simulink model "MathematicalOperations"  (R2026a)
settings: Solver=VariableStepAuto
StartFcn:
  | learning.simulink.modelCallbacks.startFunction(gcs);
StopFcn:
  | learning.simulink.modelCallbacks.stopFunction(gcs);
model workspace (MAT data in the model file):
  courseObject.course = 'simulink'
  courseObject.chapter = 4
  courseObject.lesson = 1
  courseObject.section = 1
  courseObject.task = 1
libraries: simulink x1, signalChecks x1
CloseFcn:
  | learning.simulink.cleanupOnlineTraining;learning.simulink.Application.getInstance().dduxLogMatlabEvent("ModelClosed");
Description:
  | TrainingCourseModel
settings Model: Creator=PC  LastModifiedBy=PC

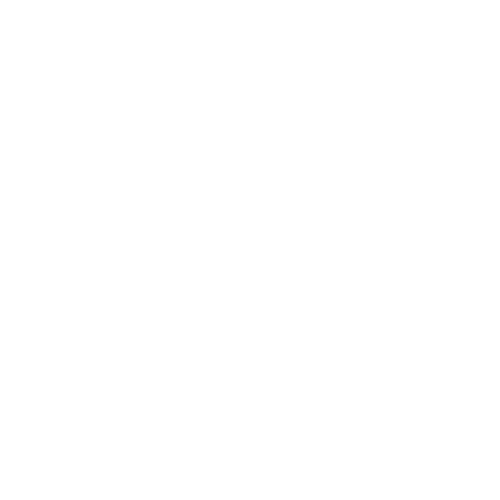
[thumbnail: Simulink's stored preview of the top-level diagram]
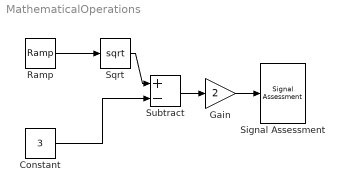
== system MathematicalOperations ==
  Constant : Constant  Value=3
  Gain : Gain  Gain=2
  Ramp : simulink/Sources/Ramp  slope=2  start=0  InitialOutput=0
  Signal Assessment : signalChecks/Signal Assessment  signal_type='signal'  t_ans=(linspace(0,10,200))'  y_ans_upper=2*(sqrt(2*linspace(0,10,200)')-3)  y_ans_lower=0  range=0.01  rate_type=0  lesson=0  task=4  pass=1
  Sqrt : Sqrt
  Subtract : Sum  Inputs=+-
  wires:
  Ramp/1 -> Sqrt/1
  Sqrt/1 -> Subtract/1
  Constant/1 -> Subtract/2
  Subtract/1 -> Gain/1
  Gain/1 -> Signal Assessment/1
